simulink library "sm_car_scene_ice_patch"  (R2026a)
settings: Solver=VariableStepAuto
undefined symbols (not defined in the file or in its folder): Scene, X, Y, Z
libraries: Scene_Utilities x3, sm_lib x1
Description:
  | Scene of Simscape Vehicle Templates Library
  | 
  | Copyright 2018-2026 The MathWorks, Inc.
settings Model: Creator=smiller  LastModifiedBy=smiller

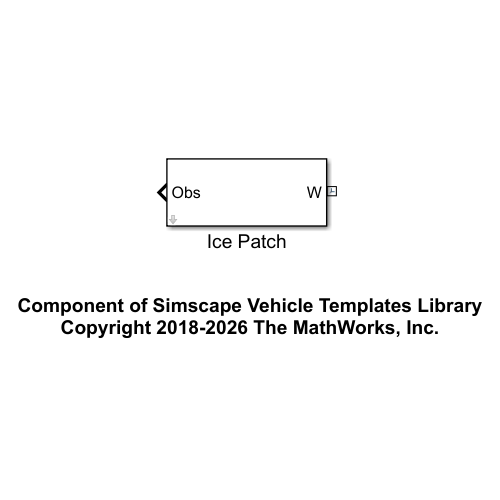
[thumbnail: Simulink's stored preview of the top-level diagram]
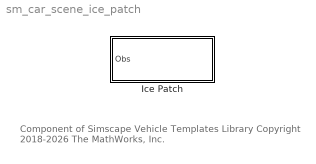
== system sm_car_scene_ice_patch ==
  note: Component of Simscape Vehicle Templates Library
      | Copyright 2018-2026 The MathWorks, Inc.
  Ice Patch : Subsystem  mask{plane=Scene.Ice_Patch.Plane, grid=Scene.Ice_Patch.Grid, ice=Scene.Ice_Patch.Ice}
      mask prompts: plane "Ground Plane (structure)"; grid "Grid (structure)"; ice "Ice Patch (structure)"

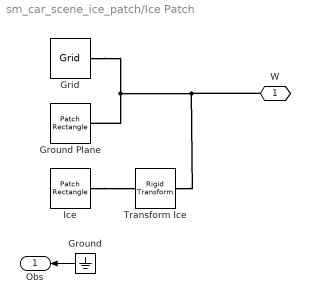
== system sm_car_scene_ice_patch/Ice Patch ==
  Grid : Scene_Utilities/Grid  grid_x=plane.l  grid_y=plane.w  grid_z=plane.h  grid_line_width=grid.line_width  grid_num_sq_x=grid.num_sqrs_x  grid_num_sq_y=grid.num_sqrs_y  grid_clr=grid.clr  grid_opc=grid.opc
  Ground : Ground
  Ground Plane : Scene_Utilities/Patch Rectangle  gp_l=plane.l  gp_w=plane.w  gp_h=plane.h  gp_clr=plane.clr  gp_opc=plane.opc
  Ice : Scene_Utilities/Patch Rectangle  gp_l=ice.x_max-ice.x_min  gp_w=ice.y_max-ice.y_min  gp_h=ice.h  gp_clr=ice.clr  gp_opc=ice.opc
  Transform Ice : sm_lib/Frames and Transforms/Rigid Transform  RotationMethod=None  FollAlignAxisA=+X  BaseAlignAxisA=+Y  FollAlignAxisB=+Y  BaseAlignAxisB=+Z  RotationStandardAxis=+Z  RotationAngle=0.0  RotationAngleUnits=deg  RotationArbitraryAxis=[0 0 1]  RotationSequenceAxes=FollowerAxes  RotationSequence=XYX  RotationSequenceAngles=[0 0 0]  RotationSequenceAnglesUnits=deg  RotationMatrix=[1 0 0; 0 1 0; 0 0 1]  Quaternion=[1 0 0 0]  TranslationMethod=Cartesian  TranslationCartesianOffset=[(ice.x_max+ice.x_min)/2,(ice.y_max+ice.y_min)/2, ice.z]  TranslationCartesianOffsetUnits=m  TranslationStandardAxis=+Z  TranslationStandardOffset=0  TranslationStandardOffsetUnits=m  TranslationROffset=0  TranslationROffsetUnits=m  TranslationThetaOffset=0  TranslationThetaOffsetUnits=deg  TranslationZOffset=0  TranslationZOffsetUnits=m
  W : PMIOPort  Side=Left
  Obs : Outport  VectorParamsAs1DForOutWhenUnconnected=off
  wires:
  Ground/1 -> Obs/1
  connections:
  Ice/RConn1 -- Transform Ice/RConn1
  Transform Ice/LConn1 -- W/RConn1 -- Grid/LConn1 -- Ground Plane/RConn1
